simulink model "snake"  (R2023a)
settings: Solver=VariableStepAuto  StartTime=0.0  StopTime=25  RelTol=1e-4  AbsTol=1e-4
InitFcn:
  | init_snake;
values from neighbouring files (symbols this model uses):
  cn = 0.5*rho*Cd*4*a*l    (= 4.6875)    [init_snake.m]
  ct = 0.5*rho*pi*Cf*(b+a)*l    (= 0.0736310778185)    [init_snake.m]
  D = fill(n,-1)    [init_snake.m]
  H = inv(In-e*e'/n)*K'    [init_snake.m]
  In = eye(n)    [init_snake.m]
  J = j*In    [init_snake.m]
  K = A'*inv(D*D')*D    [init_snake.m]
  l = 0.0625    [init_snake.m]
  lmbd1 = (1/12)*rho*pi*Cm*(a^2-b^2)^2*l^3    (= 0)    [init_snake.m]
  lmbd2 = (1/6)*rho*pi*Cf*(a+b)*l^3    (= 9.58737992429e-05)    [init_snake.m]
  lmbd3 = (1/8)*rho*pi*Cf*(a+b)*l^4    (= 4.49408433951e-06)    [init_snake.m]
  m = 0.55    [init_snake.m]
  mu_n = rho*pi*Ca*a^2*2*l    (= 0.552233083639)    [init_snake.m]
  n = 7    [init_snake.m]
  P0 = [0 ;0]    [init_snake.m]
  select = 0    [init_snake.m]
  t0 = zeros(n,1)    [init_snake.m]
  V = A'*inv(D*D')*A    [init_snake.m]
  Vx = ones(n,1)*0.1    [init_snake.m]
  Vy = ones(n,1)*0.1    [init_snake.m]
settings Model: Creator=Anton  LastModifiedBy=schfr
settings ExplorerConfigSet: InternalSimMechanicsExplorerSettings="<ExplorerConfiguration><canonicalview>default</canonicalview><AnimationSetting><BasePlaybackSpeed>1.0</BasePlaybackSpeed><PlaybackSpeedFactor>1.0</PlaybackSpeedFactor></AnimationSetting><TilePanel><TileInfo><Tiles Columns=\"1\" Count=\"1\" Rows=\"1\"><Column Weight=\"1\"/><Row Weight=\"1\"/><Tile Height=\"1\" Width=\"1\" X=\"0\" Y=\"0\"/></Tiles></TileInfo><SceneInfo><SceneViewer><BGColor><R>0.200000002980232239</R><G>0.200000002980232239</G><B>1</B></BGColor><Camera><DoPerspective>off</DoPerspective><Position><X>0.593658331578024612</X><Y>-1.48322302102350245</Y><Z>0.579318571965395046</Z></Position><Center><X>0.0143397506291000898</X><Y>-0.903904440074577709</Y><Z>-8.98352947587000017e-09</Z></Center><Up><X>-0.408248290463863073</X><Y>0.408248290463863073</Y><Z>0.816496580927726145</Z></Up><ViewLimDist>1</ViewLimDist><YLim>0.415596861547983476</YLim><XLim>0.652031825184822167</XLim></Camera></SceneViewer></SceneInfo></TilePanel><MechEditorPanel><Cameras/><GfxPanelCameraMap/><VideoCreator><PlaybackSpeedRatio>1.0</PlaybackSpeedRatio><FrameRate>30</FrameRate><VideoFormat>Motion JPEG AVI</VideoFormat><FrameSize>auto</FrameSize></VideoCreator></MechEditorPanel></ExplorerConfiguration>"

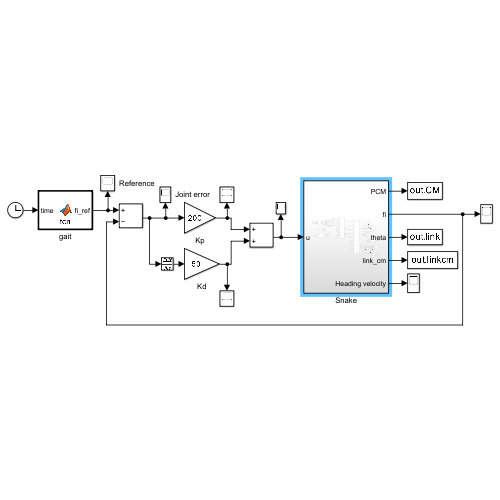
[thumbnail: Simulink's stored preview of the top-level diagram]
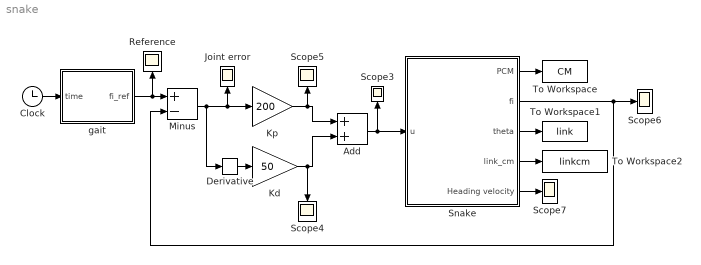
== system snake ==
  Add : Sum
  Clock : Clock
  Derivative : Derivative
  Joint error : Scope
  Kd : Gain  Gain=50
  Kp : Gain  Gain=200
  Minus : Sum  Inputs=+-
  Reference : Scope
  Scope{3..7} (5 alike) : Scope
  Snake : Subsystem
  To Workspace : ToWorkspace  VariableName=CM  SaveFormat=Timeseries  SampleTime=-1
  To Workspace1 : ToWorkspace  VariableName=link  SaveFormat=Timeseries  SampleTime=-1
  To Workspace2 : ToWorkspace  VariableName=linkcm  SaveFormat=Timeseries  SampleTime=-1
  gait : MATLAB Function  TreatAsAtomicUnit=on
  wires:
  Kp/1 -> Add/1, Scope5/1
  Derivative/1 -> Kd/1
  Add/1 -> Scope3/1, Snake/1(u)
  Minus/1 -> Kp/1, Joint error/1, Derivative/1
  gait/1(fi_ref) -> Reference/1, Minus/1
  Clock/1 -> gait/1(time)
  Kd/1 -> Add/2, Scope4/1
  Snake/3(theta) -> To Workspace1/1
  Snake/1(PCM) -> To Workspace/1
  Snake/4(link_cm) -> To Workspace2/1
  Snake/2(fi) -> Minus/2, Scope6/1
  Snake/5(Heading velocity) -> Scope7/1

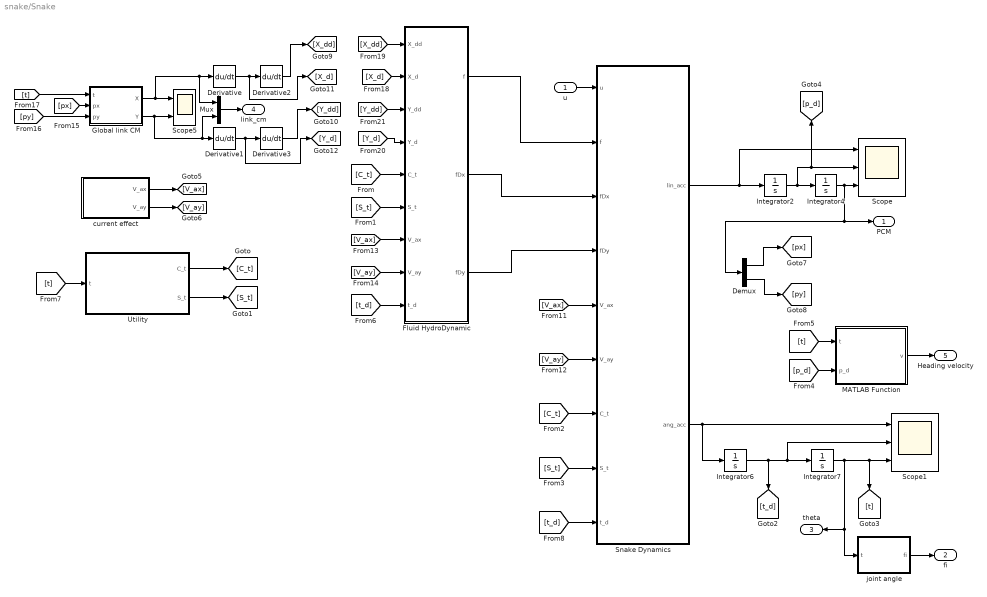
== system snake/Snake ==
  u : Inport
  Demux : Demux  Outputs=2
  Derivative{,1..3} (4 alike) : Derivative
  Fluid HydroDynamic : MATLAB Function  TreatAsAtomicUnit=on
  Global link CM : MATLAB Function  TreatAsAtomicUnit=on
  Integrator2 : Integrator  InitialCondition=P0
  Integrator4 : Integrator  InitialCondition=P0
  Integrator6 : Integrator  InitialCondition=t0
  Integrator7 : Integrator  InitialCondition=t0
  MATLAB Function : MATLAB Function  TreatAsAtomicUnit=on
  Mux : Mux  Inputs=2
  Scope : Scope  NumInputPorts=3
  Scope1 : Scope  NumInputPorts=3
  Scope5 : Scope  NumInputPorts=2
  Snake Dynamics : MATLAB Function  TreatAsAtomicUnit=on
  Utility : MATLAB Function  TreatAsAtomicUnit=on
  current effect : MATLAB Function  TreatAsAtomicUnit=on
  joint angle : MATLAB Function  TreatAsAtomicUnit=on
  PCM : Outport
  fi : Outport  Port=2
  theta : Outport  Port=3
  link_cm : Outport  Port=4
  Heading velocity : Outport  Port=5
  wires:
  Utility/1(C_t) -> [C_t]
  Fluid HydroDynamic/3(fDy) -> Snake Dynamics/4(fDy)
  Snake Dynamics/2(ang_acc) -> Scope1/1, Integrator6/1
  Utility/2(S_t) -> [S_t]
  [V_ax] -> Snake Dynamics/5(V_ax)
  Integrator6/1 -> [t_d], Integrator7/1, Scope1/2
  [t] -> Utility/1(t)
  [V_ay] -> Fluid HydroDynamic/8(V_ay)
  Fluid HydroDynamic/2(fDx) -> Snake Dynamics/3(fDx)
  [V_ay] -> Snake Dynamics/6(V_ay)
  Integrator2/1 -> Integrator4/1, [p_d], Scope/2
  [C_t] -> Fluid HydroDynamic/5(C_t)
  Fluid HydroDynamic/1(f) -> Snake Dynamics/2(f)
  [C_t] -> Snake Dynamics/7(C_t)
  [S_t] -> Snake Dynamics/8(S_t)
  current effect/1(V_ax) -> [V_ax]
  Integrator4/1 -> PCM/1, Demux/1, Scope/3
  Integrator7/1 -> [t], Scope1/3, theta/1, joint angle/1(t)
  [V_ax] -> Fluid HydroDynamic/7(V_ax)
  Snake Dynamics/1(lin_acc) -> Scope/1, Integrator2/1
  [t_d] -> Fluid HydroDynamic/9(t_d)
  [S_t] -> Fluid HydroDynamic/6(S_t)
  [t_d] -> Snake Dynamics/9(t_d)
  current effect/2(V_ay) -> [V_ay]
  u/1 -> Snake Dynamics/1(u)
  joint angle/1(fi) -> fi/1
  Demux/2 -> [py]
  Demux/1 -> [px]
  [py] -> Global link CM/3(py)
  Global link CM/2(Y) -> Derivative1/1, Mux/2, Scope5/2
  [t] -> Global link CM/1(t)
  Global link CM/1(X) -> Mux/1, Derivative/1, Scope5/1
  [px] -> Global link CM/2(px)
  Derivative/1 -> [X_d], Derivative2/1
  Derivative1/1 -> [Y_d], Derivative3/1
  Derivative2/1 -> [X_dd]
  Derivative3/1 -> [Y_dd]
  [X_d] -> Fluid HydroDynamic/2(X_d)
  [X_dd] -> Fluid HydroDynamic/1(X_dd)
  [Y_d] -> Fluid HydroDynamic/4(Y_d)
  [Y_dd] -> Fluid HydroDynamic/3(Y_dd)
  Mux/1 -> link_cm/1
  MATLAB Function/1(v) -> Heading velocity/1
  [t] -> MATLAB Function/1(t)
  [p_d] -> MATLAB Function/2(p_d)

== matlab function snake/Snake/current effect ==
  data: V_ax output; V_ay output; Vx parameter; Vy parameter
function [V_ax, V_ay] = current(Vx, Vy)

    V_ax = diag(Vx);
    V_ay = diag(Vy);

end

== matlab function snake/gait ==
  data: fi_ref output; n parameter; time input; select parameter
function fi_ref = fcn(n,time,select)

    c = 7;

    fi_ref = zeros(c-1,1);
    w = 7*pi/18;
    alpha = pi/6;
    beta = pi/6;
    gamma = 0;
    
    
    if select==0    % lateral gait
        for i=1 : n-1
            fi_ref(i) = alpha*sin(w*time + (i-1)*beta) + gamma;
        end
    end
    
    if select==1    % eel-like gait
        for i=1 : n-1
            fi_ref(i) = alpha*((n-i)/(n+1))*sin(w*time + (i-1)*beta) + gamma;
        end
    end

end

== matlab function snake/Snake/Global link CM ==
  data: t input; X output; px input; py input; Y output; l parameter; K parameter; e parameter
function [X,Y] = fcn(t,px,py,l, K, e)

    X = -l*K'*cos(t)+e*px;
    Y = -l*K'*sin(t)+e*py;

end

== matlab function snake/Snake/joint angle ==
  data: t input; fi output; n parameter
function fi = fcn(t,n)

    c = 7;
    fi = zeros(c-1,1);

    for i=1 : n-1
        fi(i) = t(i)-t(i+1);
    end

end

== matlab function snake/Snake/Fluid HydroDynamic ==
  data: X_dd input; X_d input; Y_dd input; Y_d input; C_t input; S_t input; V_ax input; V_ay input; mu_n parameter; Vx parameter; Vy parameter; ct parameter; cn parameter; t_d input; f output; fDx output; fDy output [..n]; n parameter
function [f, fDx, fDy] = HydroDynamic(X_dd, X_d, Y_dd, Y_d, C_t, S_t,V_ax,V_ay, mu_n, Vx, Vy, ct, cn, t_d,n)

    c = 7;
    
    V_r = [C_t S_t; -S_t C_t]*[X_d-Vx; Y_d-Vy];
    V_rx = V_r(1:n,:);
    V_ry = V_r(n+1:2*n,:);

    % Added mass forses
    fA = -[mu_n*S_t.^2 -mu_n*S_t*C_t; -mu_n*S_t*C_t mu_n*C_t.^2]*[X_dd; Y_dd] -... 
                  [-mu_n*S_t*C_t -mu_n*S_t.^2; mu_n*C_t.^2 mu_n*S_t*C_t]*[V_ax; V_ay]*t_d;

    % Linear drag forces
    fD1 = -[ct*C_t.^2+cn*S_t.^2 (ct-cn)*S_t*C_t; (ct-cn)*S_t*C_t ct*S_t.^2+cn*C_t.^2]*[X_d-Vx; Y_d-Vy];
    fD1x = fD1(1:n,:);
    fD1y = fD1(n+1:2*n,:); 

    % Non linear drag forces
    fD2 = [ct*C_t -cn*S_t; ct*S_t cn*C_t]*sign([V_rx; V_ry]).*[V_rx.^2; V_ry.^2];
    fD2x = fD2(1:c,:);
    fD2y = fD2(c+1:2*c,:);

    fDx = fD1x + fD2x;
    fDy = fD1y + fD2y;
    f = fA + fD1 + fD2;
end

== matlab function snake/Snake/MATLAB Function ==
  data: t input; v output; p_d input; n parameter
function v = heading(t,p_d,n)

t_sgn = 0;

for i=1 : n
    t_sgn = t_sgn + t(i,1);
end

t_sgn = t_sgn/n;

v = p_d(1,1)*cos(t_sgn) + p_d(2,1)*sin(t_sgn);


end

== matlab function snake/Snake/Snake Dynamics ==
  data: u input; f input; fDx input; fDy input; V_ax input; V_ay input; lin_acc output size=2; ang_acc output; E parameter; D parameter; C_t input; S_t input; l parameter; K parameter; lmbd3 parameter; In parameter; lmbd1 parameter; lmbd2 parameter; t_d input; J parameter; m parameter; V parameter; mu_n parameter; H parameter; n parameter
function [lin_acc, ang_acc] = Dynamics(u, f,fDx, fDy, V_ax, V_ay, E, D, C_t, S_t, l, K, lmbd3, In, lmbd1, lmbd2, t_d, J, m, V, mu_n, H,n)
    
    Lbd1 = lmbd1*In;
    Lbd2 = lmbd2*In;
    Lbd3 = lmbd3*In;
    M_t = J+m*l^2*S_t*V*S_t+m*l^2*C_t*V*C_t+Lbd1+l^2*S_t*K*mu_n*S_t.^2*H*S_t+l^2*S_t*K*mu_n*S_t*C_t*H*C_t+l^2*C_t*K*mu_n*S_t*C_t*H*S_t+l^2*C_t*K*mu_n*C_t.^2*H*C_t;
    W_t = m*l^2*S_t*V*C_t-m*l^2*C_t*V*S_t+l^2*S_t*K*mu_n*S_t.^2*H*C_t-l^2*S_t*K*mu_n*S_t*C_t*H*S_t+l^2*C_t*K*mu_n*S_t*C_t*H*C_t-l^2*C_t*K*mu_n*C_t.^2*H*S_t;
    V_t = Lbd2-l*S_t*K*mu_n*S_t*C_t*V_ax-l*S_t*K*mu_n*S_t.^2*V_ay-l*C_t*K*mu_n*C_t.^2*V_ax-l*C_t*K*mu_n*S_t*C_t*V_ay;

    lin_acc = E'*f/(n*m); 
    ang_acc = inv(M_t)*(D'*u-l*C_t*K*fDy+l*S_t*K*fDx-Lbd3*abs(t_d).*t_d-V_t*t_d-W_t*t_d.^2);
    
end

== matlab function snake/Snake/Utility ==
  data: t input; C_t output; S_t output
function [C_t, S_t] = Matrix(t)
    
   C_t = diag(cos(t));
   S_t = diag(sin(t));

end
